simulink model "ipt_velocity_sim"  (R2020b)
settings: Solver=VariableStepAuto  StartTime=0.0  StopTime=20  MaxStep=dt  RelTol=1e-3
model workspace (MATLAB code in the model file):
  | run workspace_setup_scripts/teleop_sim_setup;
undefined symbols (not defined in the file): A, active_factor, active_factor_th, b, d_T, f_0, Gamma_w, Kp_d, Kth_d, LOP_0, m, theta_tol, Ts, V, v_0, v_tol, x_0, xi_p, xi_r
libraries: simulink x12
settings Model: Creator=Shane  LastModifiedBy=shfor
settings DataIOCC: ReturnWorkspaceOutputs=off
settings DebuggingCC: PregeneratedLibrarySubsystemCodeDiagnostic=none  StrictBusMsg=WarnOnBusTreatedAsVector  ArithmeticOperatorsInVariantConditions=warning
settings SFSimCC: SimUseLocalCustomCode=off  CustomCodeUndefinedFunction=UseInterfaceOnly
settings RTWCC: RTWUseLocalCustomCode=off

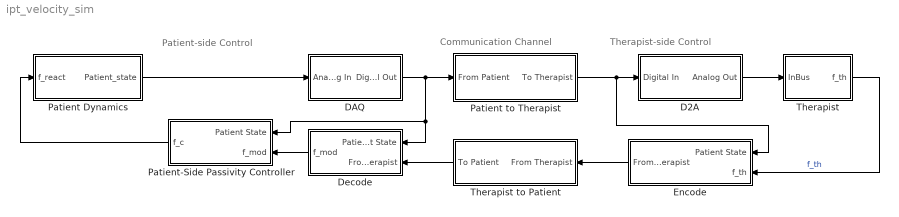
== system ipt_velocity_sim ==
  note: Patient-side Control
  note: Therapist-side Control
  note: Communication Channel
  D2A : Subsystem
  DAQ : Subsystem
  Decode : Subsystem
  Encode : Subsystem
  Patient Dynamics : Subsystem
  Patient to Therapist : Subsystem
  Patient-Side Passivity Controller : Subsystem
  Therapist : Subsystem
  Therapist to Patient : Subsystem
  wires:
  Patient-Side Passivity Controller/1(f_c) -> Patient Dynamics/1(f_react)
  Patient Dynamics/1(Patient_state) -> DAQ/1(Analog In)
  Therapist/1(f_th) -> Encode/2(f_th)  "f_th"
  Patient to Therapist/1(To Therapist) -> D2A/1(Digital In), Encode/1(Patient State)
  Encode/1(From Therapist) -> Therapist to Patient/1(From Therapist)
  Therapist to Patient/1(To Patient) -> Decode/2(From Therapist)
  Decode/1(f_mod) -> Patient-Side Passivity Controller/2(f_mod)
  DAQ/1(Digital Out) -> Patient-Side Passivity Controller/1(Patient State), Decode/1(Patient State), Patient to Therapist/1(From Patient)
  D2A/1(Analog Out) -> Therapist/1(InBus)

== system ipt_velocity_sim/D2A ==
  Digital In : Inport
  Rate Transition : RateTransition
  Analog Out : Outport  VectorParamsAs1DForOutWhenUnconnected=off
  wires:
  Digital In/1 -> Rate Transition/1
  Rate Transition/1 -> Analog Out/1

== system ipt_velocity_sim/DAQ ==
  Analog In : Inport
  Rate Transition1 : RateTransition  OutPortSampleTime=Ts
  Digital Out : Outport  VectorParamsAs1DForOutWhenUnconnected=off
  wires:
  Analog In/1 -> Rate Transition1/1
  Rate Transition1/1 -> Digital Out/1

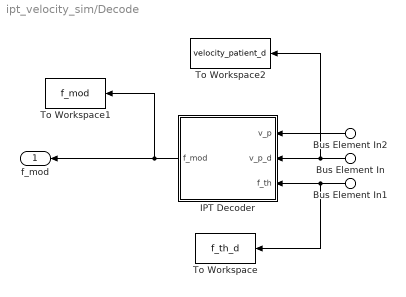
== system ipt_velocity_sim/Decode ==
  Bus Element In2 : Inport  PortName=Patient State  Element=v_p
  Bus Element In : Inport  Port=2  PortName=From Therapist  Element=v_p_d
  Bus Element In1 : Inport  Port=2  PortName=From Therapist  Element=f_th
  IPT Decoder : Subsystem  Variant=on
  To Workspace : ToWorkspace  VariableName=f_th_d  SaveFormat=Timeseries  SampleTime=-1
  To Workspace1 : ToWorkspace  VariableName=f_mod  SaveFormat=Timeseries  SampleTime=-1
  To Workspace2 : ToWorkspace  VariableName=velocity_patient_d  SaveFormat=Timeseries  SampleTime=-1
  f_mod : Outport  VectorParamsAs1DForOutWhenUnconnected=off
  wires:
  Bus Element In1/1 -> To Workspace/1, IPT Decoder/3(f_th)
  IPT Decoder/1(f_mod) -> f_mod/1, To Workspace1/1
  Bus Element In2/1 -> IPT Decoder/1(v_p)
  Bus Element In/1 -> To Workspace2/1, IPT Decoder/2(v_p_d)

== system ipt_velocity_sim/Encode ==
  In Bus Element : Inport  PortName=Patient State  Element=v_p
  f_th : Inport  Port=2
  Rate Transition1 : RateTransition  InitialCondition=f_0  OutPortSampleTime=Ts
  Out Bus Element : Outport  VectorParamsAs1DForOutWhenUnconnected=off  PortName=From Therapist  Element=v_p_d
  Out Bus Element1 : Outport  VectorParamsAs1DForOutWhenUnconnected=off  PortName=From Therapist  Element=f_th
  wires:
  f_th/1 -> Rate Transition1/1  "f_th"
  In Bus Element/1 -> Out Bus Element/1  "f_a"
  Rate Transition1/1 -> Out Bus Element1/1  "f_th"

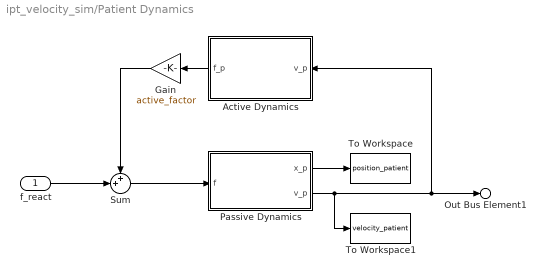
== system ipt_velocity_sim/Patient Dynamics ==
  f_react : Inport
  Active Dynamics : Subsystem
  Gain : Gain  Gain=active_factor
  Passive Dynamics : Subsystem
  Sum : Sum  Inputs=++|
  To Workspace : ToWorkspace  VariableName=position_patient  SaveFormat=Timeseries  SampleTime=-1
  To Workspace1 : ToWorkspace  VariableName=velocity_patient  SaveFormat=Timeseries  SampleTime=-1
  Out Bus Element1 : Outport  VectorParamsAs1DForOutWhenUnconnected=off  PortName=Patient_state  Element=v_p
  wires:
  Passive Dynamics/1(x_p) -> To Workspace/1
  Passive Dynamics/2(v_p) -> Out Bus Element1/1, Active Dynamics/1(v_p), To Workspace1/1
  f_react/1 -> Sum/2
  Sum/1 -> Passive Dynamics/1(f)
  Active Dynamics/1(f_p) -> Gain/1
  Gain/1 -> Sum/1

== system ipt_velocity_sim/Patient to Therapist ==
  From Patient : Inport
  Delay : Delay  DelayLength=d_T
  To Therapist : Outport  VectorParamsAs1DForOutWhenUnconnected=off
  wires:
  From Patient/1 -> Delay/1
  Delay/1 -> To Therapist/1

== system ipt_velocity_sim/Patient-Side Passivity Controller ==
  Bus Element In2 : Inport  PortName=Patient State  Element=v_p
  f_mod : Inport  Port=2
  Control Selection (Variant) : Subsystem  Variant=on
  Rate Transition : RateTransition
  f_c : Outport
  wires:
  Rate Transition/1 -> f_c/1
  f_mod/1 -> Control Selection (Variant)/1(f_mod)
  Control Selection (Variant)/1(f_c) -> Rate Transition/1
  Bus Element In2/1 -> Control Selection (Variant)/2(v_p)

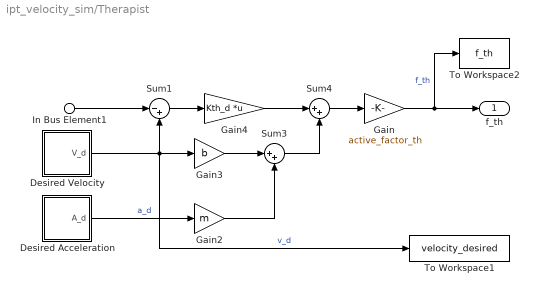
== system ipt_velocity_sim/Therapist ==
  In Bus Element1 : Inport  PortName=InBus  Element=v_p
  Desired Acceleration : Subsystem
  Desired Velocity : Subsystem
  Gain : Gain  Gain=active_factor_th
  Gain2 : Gain  Gain=m
  Gain3 : Gain  Gain=b
  Gain4 : Gain  Gain=Kth_d  Multiplication=Matrix(K*u)
  Sum1 : Sum  Inputs=|-+
  Sum3 : Sum  Inputs=|++
  Sum4 : Sum  Inputs=|++
  To Workspace1 : ToWorkspace  VariableName=velocity_desired  SaveFormat=Timeseries  SampleTime=-1
  To Workspace2 : ToWorkspace  VariableName=f_th  SaveFormat=Timeseries  SampleTime=-1
  f_th : Outport  VectorParamsAs1DForOutWhenUnconnected=off
  wires:
  Desired Velocity/1(V_d) -> To Workspace1/1, Sum1/2, Gain3/1  "v_d"
  Desired Acceleration/1(A_d) -> Gain2/1  "a_d"
  Gain3/1 -> Sum3/1
  Gain2/1 -> Sum3/2
  Sum4/1 -> Gain/1
  In Bus Element1/1 -> Sum1/1
  Sum1/1 -> Gain4/1
  Sum3/1 -> Sum4/2
  Gain4/1 -> Sum4/1
  Gain/1 -> f_th/1, To Workspace2/1  "f_th"

== system ipt_velocity_sim/Therapist to Patient ==
  From Therapist : Inport
  Delay : Delay  DelayLength=d_T
  To Patient : Outport  VectorParamsAs1DForOutWhenUnconnected=off
  wires:
  From Therapist/1 -> Delay/1
  Delay/1 -> To Patient/1

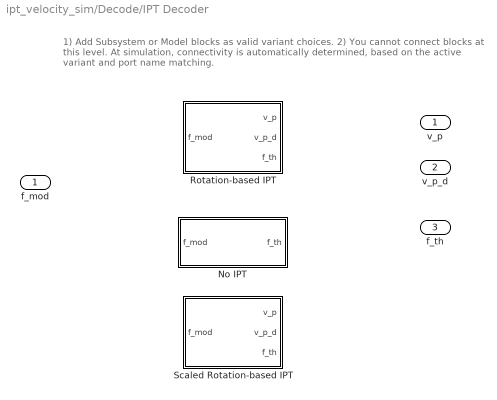
== system ipt_velocity_sim/Decode/IPT Decoder ==
  note: 1) Add Subsystem or Model blocks as valid variant choices.
      | 2) You cannot connect blocks at this level. At simulation, connectivity is automatically
      | determined, based on the active variant and port name matching.
  v_p : Inport
  v_p_d : Inport  Port=2
  f_th : Inport  Port=3
  No IPT : Subsystem  VariantControl=(default)
  Rotation-based IPT : Subsystem  VariantControl=rotationIPT
  Scaled Rotation-based IPT : Subsystem  VariantControl=scaledRIPT
  f_mod : Outport

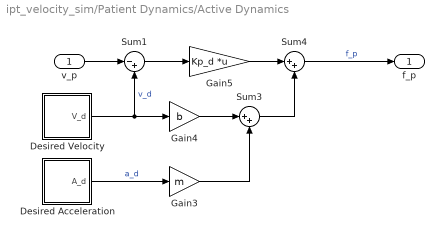
== system ipt_velocity_sim/Patient Dynamics/Active Dynamics ==
  v_p : Inport
  Desired Acceleration : Subsystem
  Desired Velocity : Subsystem
  Gain3 : Gain  Gain=m
  Gain4 : Gain  Gain=b
  Gain5 : Gain  Gain=Kp_d  Multiplication=Matrix(K*u)
  Sum1 : Sum  Inputs=|-+
  Sum3 : Sum  Inputs=|++
  Sum4 : Sum  Inputs=|++
  f_p : Outport
  wires:
  Sum4/1 -> f_p/1  "f_p"
  Sum3/1 -> Sum4/2
  Desired Velocity/1(V_d) -> Sum1/2, Gain4/1  "v_d"
  Gain5/1 -> Sum4/1
  Gain3/1 -> Sum3/2
  Gain4/1 -> Sum3/1
  Desired Acceleration/1(A_d) -> Gain3/1  "a_d"
  Sum1/1 -> Gain5/1
  v_p/1 -> Sum1/1

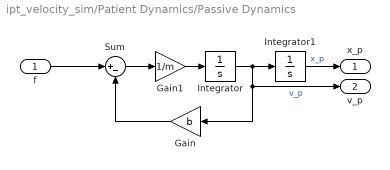
== system ipt_velocity_sim/Patient Dynamics/Passive Dynamics ==
  f : Inport
  Gain : Gain  Gain=b
  Gain1 : Gain  Gain=1/m
  Integrator : Integrator  InitialCondition=v_0
  Integrator1 : Integrator  InitialCondition=x_0
  Sum : Sum  Inputs=|+-
  x_p : Outport
  v_p : Outport  Port=2
  wires:
  f/1 -> Sum/1
  Gain1/1 -> Integrator/1
  Integrator/1 -> v_p/1, Gain/1, Integrator1/1  "v_p"
  Sum/1 -> Gain1/1
  Integrator1/1 -> x_p/1  "x_p"
  Gain/1 -> Sum/2

== system ipt_velocity_sim/Patient-Side Passivity Controller/Control Selection (Variant) ==
  note: 1) Add Subsystem or Model blocks as valid variant choices.
      | 2) You cannot connect blocks at this level. At simulation, connectivity is automatically
      | determined, based on the active variant and port name matching.
  f_mod : Inport
  v_p : Inport  Port=2
  M-TDPC : Subsystem  VariantControl=mtdpc_patient
  No Control : Subsystem  VariantControl=(default)
  f_c : Outport

== system ipt_velocity_sim/Therapist/Desired Acceleration ==
  Mux : Mux  Inputs=3
  X Acceleration : simulink/Sources/Repeating Sequence  rep_seq_t=t  rep_seq_y=A(1,:)
  Y Acceleration : simulink/Sources/Repeating Sequence  rep_seq_t=t  rep_seq_y=A(2,:)
  Z Acceleration : simulink/Sources/Repeating Sequence  rep_seq_t=t  rep_seq_y=A(3,:)
  A_d : Outport
  wires:
  Z Acceleration/1 -> Mux/3
  Y Acceleration/1 -> Mux/2
  X Acceleration/1 -> Mux/1
  Mux/1 -> A_d/1

== system ipt_velocity_sim/Therapist/Desired Velocity ==
  Mux : Mux  Inputs=3
  X Velocity : simulink/Sources/Repeating Sequence  rep_seq_t=t  rep_seq_y=V(1,:)
  Y Velocity : simulink/Sources/Repeating Sequence  rep_seq_t=t  rep_seq_y=V(2,:)
  Z Velocity : simulink/Sources/Repeating Sequence  rep_seq_t=t  rep_seq_y=V(3,:)
  V_d : Outport
  wires:
  Mux/1 -> V_d/1
  X Velocity/1 -> Mux/1
  Y Velocity/1 -> Mux/2
  Z Velocity/1 -> Mux/3

== system ipt_velocity_sim/Decode/IPT Decoder/No IPT ==
  f_th : Inport
  f_mod : Outport
  wires:
  f_th/1 -> f_mod/1

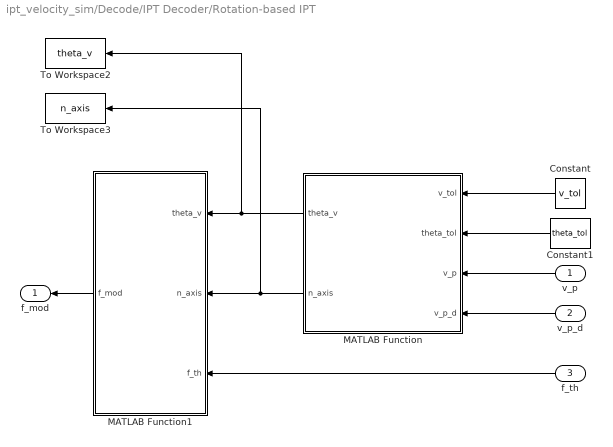
== system ipt_velocity_sim/Decode/IPT Decoder/Rotation-based IPT ==
  v_p : Inport
  v_p_d : Inport  Port=2
  f_th : Inport  Port=3
  Constant : Constant  Value=v_tol
  Constant1 : Constant  Value=theta_tol
  MATLAB Function : MATLAB Function  TreatAsAtomicUnit=on
  MATLAB Function1 : MATLAB Function  TreatAsAtomicUnit=on
  To Workspace2 : ToWorkspace  VariableName=theta_v  SaveFormat=Timeseries  SampleTime=-1
  To Workspace3 : ToWorkspace  VariableName=n_axis  SaveFormat=Timeseries  SampleTime=-1
  f_mod : Outport
  wires:
  Constant/1 -> MATLAB Function/1(v_tol)
  MATLAB Function/1(theta_v) -> MATLAB Function1/1(theta_v), To Workspace2/1
  Constant1/1 -> MATLAB Function/2(theta_tol)
  MATLAB Function/2(n_axis) -> To Workspace3/1, MATLAB Function1/2(n_axis)
  MATLAB Function1/1(f_mod) -> f_mod/1
  v_p/1 -> MATLAB Function/3(v_p)
  v_p_d/1 -> MATLAB Function/4(v_p_d)
  f_th/1 -> MATLAB Function1/3(f_th)

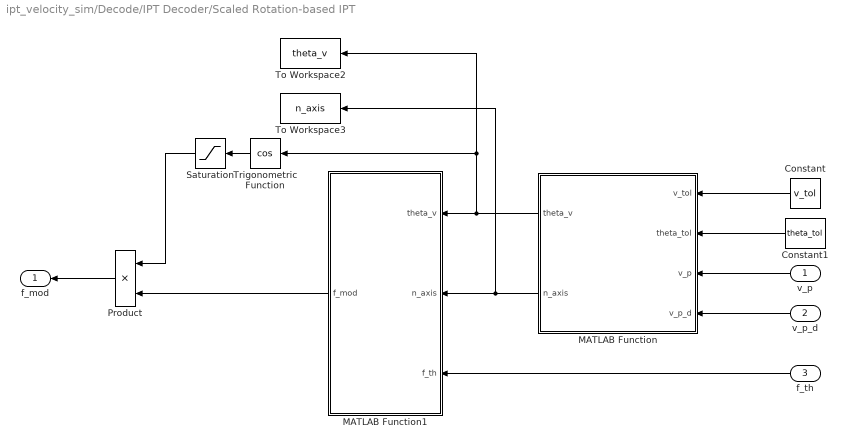
== system ipt_velocity_sim/Decode/IPT Decoder/Scaled Rotation-based IPT ==
  v_p : Inport
  v_p_d : Inport  Port=2
  f_th : Inport  Port=3
  Constant : Constant  Value=v_tol
  Constant1 : Constant  Value=theta_tol
  MATLAB Function : MATLAB Function  TreatAsAtomicUnit=on
  MATLAB Function1 : MATLAB Function  TreatAsAtomicUnit=on
  Product : Product
  Saturation : Saturate  UpperLimit=1  LowerLimit=0
  To Workspace2 : ToWorkspace  VariableName=theta_v  SaveFormat=Timeseries  SampleTime=-1
  To Workspace3 : ToWorkspace  VariableName=n_axis  SaveFormat=Timeseries  SampleTime=-1
  Trigonometric Function : Trigonometry  Operator=cos
  f_mod : Outport
  wires:
  Constant/1 -> MATLAB Function/1(v_tol)
  MATLAB Function/1(theta_v) -> MATLAB Function1/1(theta_v), To Workspace2/1, Trigonometric Function/1
  Constant1/1 -> MATLAB Function/2(theta_tol)
  MATLAB Function/2(n_axis) -> To Workspace3/1, MATLAB Function1/2(n_axis)
  v_p/1 -> MATLAB Function/3(v_p)
  v_p_d/1 -> MATLAB Function/4(v_p_d)
  f_th/1 -> MATLAB Function1/3(f_th)
  Trigonometric Function/1 -> Saturation/1
  MATLAB Function1/1(f_mod) -> Product/2
  Product/1 -> f_mod/1
  Saturation/1 -> Product/1

== system ipt_velocity_sim/Patient Dynamics/Active Dynamics/Desired Acceleration ==
  Mux : Mux  Inputs=3
  X Acceleration : simulink/Sources/Repeating Sequence  rep_seq_t=t  rep_seq_y=A(1,:)
  Y Acceleration : simulink/Sources/Repeating Sequence  rep_seq_t=t  rep_seq_y=A(2,:)
  Z Acceleration : simulink/Sources/Repeating Sequence  rep_seq_t=t  rep_seq_y=A(3,:)
  A_d : Outport
  wires:
  Z Acceleration/1 -> Mux/3
  Y Acceleration/1 -> Mux/2
  X Acceleration/1 -> Mux/1
  Mux/1 -> A_d/1

== system ipt_velocity_sim/Patient Dynamics/Active Dynamics/Desired Velocity ==
  Mux : Mux  Inputs=3
  X Velocity : simulink/Sources/Repeating Sequence  rep_seq_t=t  rep_seq_y=V(1,:)
  Y Velocity : simulink/Sources/Repeating Sequence  rep_seq_t=t  rep_seq_y=V(2,:)
  Z Velocity : simulink/Sources/Repeating Sequence  rep_seq_t=t  rep_seq_y=V(3,:)
  V_d : Outport
  wires:
  Mux/1 -> V_d/1
  X Velocity/1 -> Mux/1
  Y Velocity/1 -> Mux/2
  Z Velocity/1 -> Mux/3

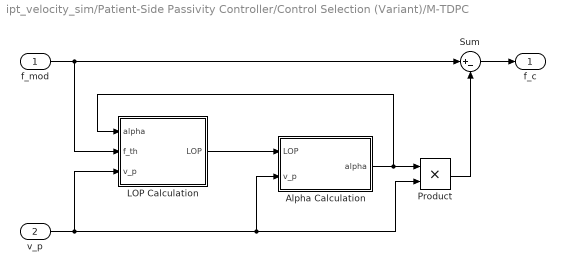
== system ipt_velocity_sim/Patient-Side Passivity Controller/Control Selection (Variant)/M-TDPC ==
  f_mod : Inport
  v_p : Inport  Port=2
  Alpha Calculation : Subsystem
  LOP Calculation : Subsystem
  Product : Product
  Sum : Sum  Inputs=|+-
  f_c : Outport
  wires:
  Sum/1 -> f_c/1
  f_mod/1 -> Sum/1, LOP Calculation/2(f_th)
  v_p/1 -> LOP Calculation/3(v_p), Alpha Calculation/2(v_p), Product/2
  Alpha Calculation/1(alpha) -> Product/1, LOP Calculation/1(alpha)
  Product/1 -> Sum/2
  LOP Calculation/1(LOP) -> Alpha Calculation/1(LOP)

== system ipt_velocity_sim/Patient-Side Passivity Controller/Control Selection (Variant)/No Control ==
  f_mod : Inport
  f_c : Outport
  wires:
  f_mod/1 -> f_c/1

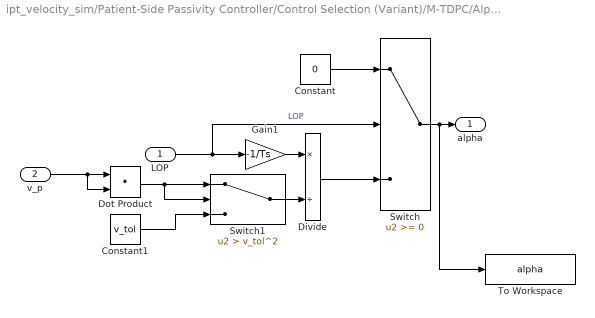
== system ipt_velocity_sim/Patient-Side Passivity Controller/Control Selection (Variant)/M-TDPC/Alpha Calculation ==
  LOP : Inport
  v_p : Inport  Port=2
  Constant : Constant  Value=0
  Constant1 : Constant  Value=v_tol
  Divide : Product  Inputs=*/
  Dot Product : DotProduct  InputSameDT=on  OutDataTypeStr=Inherit: Inherit via internal rule
  Gain1 : Gain  Gain=-1/Ts
  Switch : Switch
  Switch1 : Switch  Criteria=u2 > Threshold  Threshold=v_tol^2
  To Workspace : ToWorkspace  VariableName=alpha  SaveFormat=Timeseries  SampleTime=-1
  alpha : Outport
  wires:
  Constant/1 -> Switch/1
  Divide/1 -> Switch/3
  Gain1/1 -> Divide/1
  LOP/1 -> Gain1/1, Switch/2  "LOP"
  v_p/1 -> Dot Product/2, Dot Product/1
  Switch1/1 -> Divide/2
  Dot Product/1 -> Switch1/2, Switch1/1
  Constant1/1 -> Switch1/3
  Switch/1 -> To Workspace/1, alpha/1

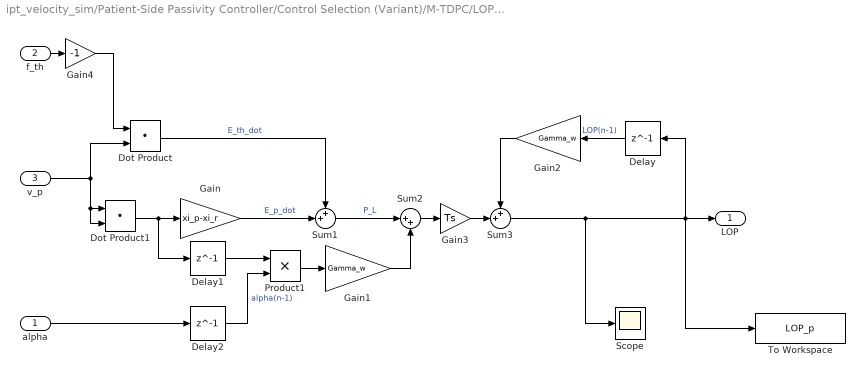
== system ipt_velocity_sim/Patient-Side Passivity Controller/Control Selection (Variant)/M-TDPC/LOP Calculation ==
  alpha : Inport
  f_th : Inport  Port=2
  v_p : Inport  Port=3
  Delay : Delay  DelayLength=1  InitialCondition=LOP_0
  Delay1 : Delay  DelayLength=1
  Delay2 : Delay  DelayLength=1
  Dot Product : DotProduct  InputSameDT=on  OutDataTypeStr=Inherit: Inherit via internal rule
  Dot Product1 : DotProduct  InputSameDT=on  OutDataTypeStr=Inherit: Inherit via internal rule
  Gain : Gain  Gain=xi_p-xi_r
  Gain1 : Gain  Gain=Gamma_w
  Gain2 : Gain  Gain=Gamma_w
  Gain3 : Gain  Gain=Ts
  Gain4 : Gain  Gain=-1
  Product1 : Product
  Scope : Scope
  Sum1 : Sum  Inputs=++|
  Sum2 : Sum  Inputs=|++
  Sum3 : Sum  Inputs=++|
  To Workspace : ToWorkspace  VariableName=LOP_p  SaveFormat=Timeseries  SampleTime=-1
  LOP : Outport
  wires:
  Sum2/1 -> Gain3/1
  Gain/1 -> Sum1/2  "E_p_dot"
  Delay/1 -> Gain2/1  "LOP(n-1)"
  Dot Product/1 -> Sum1/1  "E_th_dot"
  Delay1/1 -> Product1/1
  Dot Product1/1 -> Delay1/1, Gain/1
  alpha/1 -> Delay2/1
  Sum3/1 -> Scope/1, To Workspace/1, LOP/1, Delay/1
  Product1/1 -> Gain1/1
  Delay2/1 -> Product1/2  "alpha(n-1)"
  Gain2/1 -> Sum3/1
  Gain1/1 -> Sum2/2
  Sum1/1 -> Sum2/1  "P_L"
  Gain3/1 -> Sum3/2
  v_p/1 -> Dot Product1/2, Dot Product1/1, Dot Product/2
  f_th/1 -> Gain4/1
  Gain4/1 -> Dot Product/1

== matlab function ipt_velocity_sim/Decode/IPT Decoder/Rotation-based IPT/MATLAB Function1 ==
  data: theta_v input; f_mod output; n_axis input; f_th input
function f_mod = rotate_vector(theta_v, n_axis, f_th)

f_mod = axis_angle_rotate(n_axis, theta_v, f_th);

== matlab function ipt_velocity_sim/Decode/IPT Decoder/Rotation-based IPT/MATLAB Function ==
  data: v_tol input; theta_tol input; v_p input; theta_v output; v_p_d input; n_axis output
function [theta_v, n_axis] = calc_angle_axis(v_tol, theta_tol, v_p, v_p_d)
% CALC_ANGLE_AXIS Calculates the relative angle-axis rotation between vectors
%   [theta_v, n_axis] = calc_angle_axis(v_tol, theta_tol, v_p, v_p_d)
%   Calculates the angle and axis describing the rotation between two
%   vectors. If either of the vectors are smaller than v_tol the rotation
%   is not well defined and the function outputs default no-rotation
%   values. If the angle is very small, the axis is not well-defined, so
%   the function outputs the default no-rotation value.

% Default outputs (no rotation)
theta_v = 0;
n_axis = zeros(size(v_p));
n_axis(end) = 1;

v_p_mag = norm(v_p);
v_p_d_mag = norm(v_p_d);

if v_p_mag > v_tol && v_p_d_mag > v_tol
    theta_v = acos(dot(v_p,v_p_d)/(v_p_mag*v_p_d_mag));
    if theta_v > theta_tol
        n_axis = cross(v_p_d, v_p)/(v_p_mag*v_p_d_mag*sin(theta_v));
    else
        theta_v = 0;
    end
end

== matlab function ipt_velocity_sim/Decode/IPT Decoder/Scaled Rotation-based IPT/MATLAB Function ==
  data: v_tol input; theta_tol input; v_p input; theta_v output; v_p_d input; n_axis output
function [theta_v, n_axis] = calc_angle_axis(v_tol, theta_tol, v_p, v_p_d)
% CALC_ANGLE_AXIS Calculates the relative angle-axis rotation between vectors
%   [theta_v, n_axis] = calc_angle_axis(v_tol, theta_tol, v_p, v_p_d)
%   Calculates the angle and axis describing the rotation between two
%   vectors. If either of the vectors are smaller than v_tol the rotation
%   is not well defined and the function outputs default no-rotation
%   values. If the angle is very small, the axis is not well-defined, so
%   the function outputs the default no-rotation value.

% Default outputs (no rotation)
theta_v = 0;
n_axis = zeros(size(v_p));
n_axis(end) = 1;

v_p_mag = norm(v_p);
v_p_d_mag = norm(v_p_d);

if v_p_mag > v_tol && v_p_d_mag > v_tol
    theta_v = acos(dot(v_p,v_p_d)/(v_p_mag*v_p_d_mag));
    if theta_v > theta_tol
        n_axis = cross(v_p_d, v_p)/(v_p_mag*v_p_d_mag*sin(theta_v));
    else
        theta_v = 0;
    end
end

== matlab function ipt_velocity_sim/Decode/IPT Decoder/Scaled Rotation-based IPT/MATLAB Function1 ==
  data: theta_v input; f_mod output; n_axis input; f_th input
function f_mod = rotate_vector(theta_v, n_axis, f_th)

f_mod = axis_angle_rotate(n_axis, theta_v, f_th);
